simulink model "rocket"  (R2020a)
settings: Solver=FixedStepAuto  StartTime=0.0  StopTime=60  FixedStep=.1  RelTol=1e-3
InitFcn:
  | init
StopFcn:
  | plot_results
values from neighbouring files (symbols this model uses):
  d0 = 10    [init.m]
  d1 = 1    [init.m]
  F = 2*M*g    (= 21777.7777778)    [init.m]
  g = 9.8    [init.m]
  Ib = 1/4*mb*d1^2 + 1/12*mb*(2*d0)^2    (= 33583.3333333)    [init.m]
  M = mb + mc    (= 1111.11111111)    [init.m]
  mb = 1000    [init.m]
  mc = p/(1-p)*mb    (= 111.111111111)    [init.m]
  theta_ref = 10*pi/180    (= 0.174532925199)    [init.m]    (also in plot_results.m = out.theta_ref.Data)
libraries: simulink x2
settings Model: Creator=Tyler  LastModifiedBy=Tyler

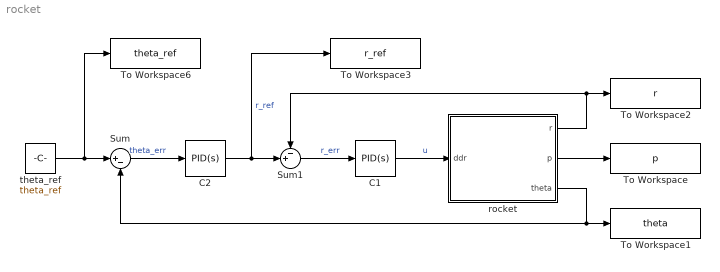
== system rocket ==
  C1 : simulink/Continuous/PID Controller  Controller=PID  Form=Parallel  TimeDomain=Continuous-time  UseExternalTs=off  SampleTime=-1  IntegratorMethod=Forward Euler  FilterMethod=Forward Euler  ControllerParametersSource=internal  P=30.7871197003863  I=15.2855535530538  D=10.7168713774137  UseFilter=on  N=29.8149109902028  TunerSelectOption=Transfer Function Based (PID Tuner App)  InitialConditionSource=internal  InitialConditionForIntegrator=0  InitialConditionForFilter=0  DifferentiatorICPrevScaledInput=0  ExternalReset=none  TrackingMode=off  Kt=1  LimitOutput=off  UpperSaturationLimit=inf  LowerSaturationLimit=-inf  LinearizeAsGain=on  AntiWindupMode=none  Kb=1  POutMin=[]  POutMax=[]  IOutMin=[]  IOutMax=[]  DOutMin=[]  DOutMax=[]  NOutMin=[]  NOutMax=[]  SumOutMin=[]  SumOutMax=[]  SaturationOutMin=[]  SaturationOutMax=[]  PParamMin=[]  PParamMax=[]  IParamMin=[]  IParamMax=[]  DParamMin=[]  DParamMax=[]  NParamMin=[]  NParamMax=[]  KbParamMin=[]  KbParamMax=[]  KtParamMin=[]  KtParamMax=[]  KbOutMin=[]  KbOutMax=[]  KtOutMin=[]  KtOutMax=[]  IntegratorOutMin=[]  IntegratorOutMax=[]  FilterOutMin=[]  FilterOutMax=[]  SumI1OutMin=[]  SumI1OutMax=[]  SumI2OutMin=[]  SumI2OutMax=[]  SumI3OutMin=[]  SumI3OutMax=[]  SumI4OutMin=[]  SumI4OutMax=[]  SumDOutMin=[]  SumDOutMax=[]  DifferentiatorOutMin=[]  DifferentiatorOutMax=[]  FilterDiffOutCoefMin=[]  FilterDiffOutCoefMax=[]  ReciprocalOutMin=[]  ReciprocalOutMax=[]  SumDenOutMin=[]  SumDenOutMax=[]  SumNumOutMin=[]  SumNumOutMax=[]  DivideOutMin=[]  DivideOutMax=[]  UdiffTsProdOutMin=[]  UdiffTsProdOutMax=[]  NTsProdOutMin=[]  NTsProdOutMax=[]  UintegralTsProdOutMin=[]  UintegralTsProdOutMax=[]  UngainTsProdOutMin=[]  UngainTsProdOutMax=[]  IntegratorContinuousStateAttributes=''  IntegratorStateMustResolveToSignalObject=off  IntegratorRTWStateStorageClass=Auto  FilterContinuousStateAttributes=''  FilterStateMustResolveToSignalObject=off  FilterRTWStateStorageClass=Auto  ParallelPVariant=InternalParameters  IdealPVariant=Disabled  IVariant=InternalParameters  DVariant=InternalParameters  IntegratorVariant=Continuous  SatVariant=Disabled  AWVariant=Passthrough  PCopyVariant=Disabled  TRVariant=Disabled  FdbkBlocksVariant=Forward  IdealPFdbkVariant=Disabled  SatFdbkVariant=Disabled  DerivativeFilterVariant=ContFilter  NVariant=InternalParameters  NCopyVariant=Disabled  FilterICVariant=InternalICsFilter  IntegratorICVariant=InternalICs  ExternalResetVariant=Disabled  TRSumVariant=Passthrough  SumFdbkVariant=Disabled  SumVariant=Sum_PID  TsampFilterVariant=InternalTs  TsampNgainVariant=Passthrough  TsampIntegralVariant=Passthrough
  C2 : simulink/Continuous/PID Controller  Controller=PID  Form=Parallel  TimeDomain=Continuous-time  UseExternalTs=off  SampleTime=-1  IntegratorMethod=Forward Euler  FilterMethod=Forward Euler  ControllerParametersSource=internal  P=0.486154115731224  I=0.0253600241547768  D=2.20545552139545  UseFilter=on  N=2.12291335792304  TunerSelectOption=Transfer Function Based (PID Tuner App)  InitialConditionSource=internal  InitialConditionForIntegrator=0  InitialConditionForFilter=0  DifferentiatorICPrevScaledInput=0  ExternalReset=none  TrackingMode=off  Kt=1  LimitOutput=off  UpperSaturationLimit=inf  LowerSaturationLimit=-inf  LinearizeAsGain=on  AntiWindupMode=none  Kb=1  POutMin=[]  POutMax=[]  IOutMin=[]  IOutMax=[]  DOutMin=[]  DOutMax=[]  NOutMin=[]  NOutMax=[]  SumOutMin=[]  SumOutMax=[]  SaturationOutMin=[]  SaturationOutMax=[]  PParamMin=[]  PParamMax=[]  IParamMin=[]  IParamMax=[]  DParamMin=[]  DParamMax=[]  NParamMin=[]  NParamMax=[]  KbParamMin=[]  KbParamMax=[]  KtParamMin=[]  KtParamMax=[]  KbOutMin=[]  KbOutMax=[]  KtOutMin=[]  KtOutMax=[]  IntegratorOutMin=[]  IntegratorOutMax=[]  FilterOutMin=[]  FilterOutMax=[]  SumI1OutMin=[]  SumI1OutMax=[]  SumI2OutMin=[]  SumI2OutMax=[]  SumI3OutMin=[]  SumI3OutMax=[]  SumI4OutMin=[]  SumI4OutMax=[]  SumDOutMin=[]  SumDOutMax=[]  DifferentiatorOutMin=[]  DifferentiatorOutMax=[]  FilterDiffOutCoefMin=[]  FilterDiffOutCoefMax=[]  ReciprocalOutMin=[]  ReciprocalOutMax=[]  SumDenOutMin=[]  SumDenOutMax=[]  SumNumOutMin=[]  SumNumOutMax=[]  DivideOutMin=[]  DivideOutMax=[]  UdiffTsProdOutMin=[]  UdiffTsProdOutMax=[]  NTsProdOutMin=[]  NTsProdOutMax=[]  UintegralTsProdOutMin=[]  UintegralTsProdOutMax=[]  UngainTsProdOutMin=[]  UngainTsProdOutMax=[]  IntegratorContinuousStateAttributes=''  IntegratorStateMustResolveToSignalObject=off  IntegratorRTWStateStorageClass=Auto  FilterContinuousStateAttributes=''  FilterStateMustResolveToSignalObject=off  FilterRTWStateStorageClass=Auto  ParallelPVariant=InternalParameters  IdealPVariant=Disabled  IVariant=InternalParameters  DVariant=InternalParameters  IntegratorVariant=Continuous  SatVariant=Disabled  AWVariant=Passthrough  PCopyVariant=Disabled  TRVariant=Disabled  FdbkBlocksVariant=Forward  IdealPFdbkVariant=Disabled  SatFdbkVariant=Disabled  DerivativeFilterVariant=ContFilter  NVariant=InternalParameters  NCopyVariant=Disabled  FilterICVariant=InternalICsFilter  IntegratorICVariant=InternalICs  ExternalResetVariant=Disabled  TRSumVariant=Passthrough  SumFdbkVariant=Disabled  SumVariant=Sum_PID  TsampFilterVariant=InternalTs  TsampNgainVariant=Passthrough  TsampIntegralVariant=Passthrough
  Sum : Sum  Inputs=|+-
  Sum1 : Sum  Inputs=-+|
  To Workspace : ToWorkspace  VariableName=p  SaveFormat=Timeseries  SampleTime=-1
  To Workspace1 : ToWorkspace  VariableName=theta  SaveFormat=Timeseries  SampleTime=-1
  To Workspace2 : ToWorkspace  VariableName=r  SaveFormat=Timeseries  SampleTime=-1
  To Workspace3 : ToWorkspace  VariableName=r_ref  SaveFormat=Timeseries  SampleTime=-1
  To Workspace6 : ToWorkspace  VariableName=theta_ref  SaveFormat=Timeseries  SampleTime=-1
  rocket : Subsystem
  theta_ref : Constant  Value=theta_ref
  wires:
  Sum1/1 -> C1/1  "r_err"
  rocket/3(theta) -> To Workspace1/1, Sum/2
  C1/1 -> rocket/1(ddr)  "u"
  rocket/1(r) -> To Workspace2/1, Sum1/1
  rocket/2(p) -> To Workspace/1
  Sum/1 -> C2/1  "theta_err"
  C2/1 -> To Workspace3/1, Sum1/2  "r_ref"
  theta_ref/1 -> To Workspace6/1, Sum/1

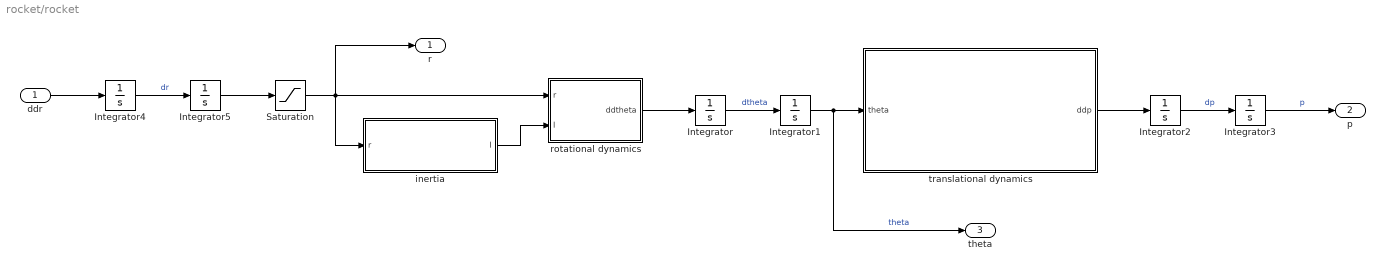
== system rocket/rocket ==
  ddr : Inport
  Integrator{,1..5} (6 alike) : Integrator
  Saturation : Saturate  UpperLimit=1  LowerLimit=-1
  inertia : Subsystem
  rotational dynamics : Subsystem
  translational dynamics : Subsystem
  r : Outport
  p : Outport  Port=2
  theta : Outport  Port=3
  wires:
  Integrator5/1 -> Saturation/1
  Integrator/1 -> Integrator1/1  "dtheta"
  inertia/1(I) -> rotational dynamics/2(I)
  rotational dynamics/1(ddtheta) -> Integrator/1
  Integrator4/1 -> Integrator5/1  "dr"
  Integrator2/1 -> Integrator3/1  "dp"
  Integrator3/1 -> p/1  "p"
  translational dynamics/1(ddp) -> Integrator2/1
  ddr/1 -> Integrator4/1
  Saturation/1 -> r/1, rotational dynamics/1(r), inertia/1(r)
  Integrator1/1 -> theta/1, translational dynamics/1(theta)  "theta"

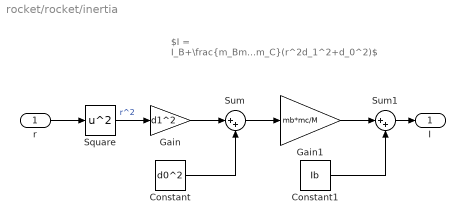
== system rocket/rocket/inertia ==
  note: $I = I_B+\frac{m_Bm_C}{m_B+m_C}(r^2d_1^2+d_0^2)$
  r : Inport
  Constant : Constant  Value=d0^2
  Constant1 : Constant  Value=Ib
  Gain : Gain  Gain=d1^2
  Gain1 : Gain  Gain=mb*mc/M
  Square : Math  Operator=square  SaturateOnIntegerOverflow=on
  Sum : Sum  Inputs=|++
  Sum1 : Sum  Inputs=|++
  I : Outport
  wires:
  Gain/1 -> Sum/1
  Gain1/1 -> Sum1/1
  Constant/1 -> Sum/2
  Constant1/1 -> Sum1/2
  Square/1 -> Gain/1  "r^2"
  Sum/1 -> Gain1/1
  r/1 -> Square/1
  Sum1/1 -> I/1

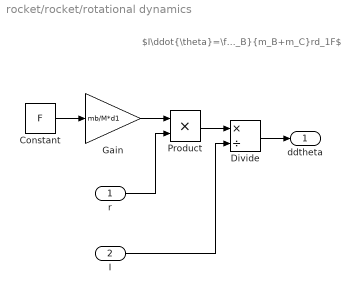
== system rocket/rocket/rotational dynamics ==
  note: $I\ddot{\theta}=\frac{m_B}{m_B+m_C}rd_1F$
  r : Inport
  I : Inport  Port=2
  Constant : Constant  Value=F
  Divide : Product  Inputs=*/
  Gain : Gain  Gain=mb/M*d1
  Product : Product
  ddtheta : Outport
  wires:
  Divide/1 -> ddtheta/1
  I/1 -> Divide/2
  Constant/1 -> Gain/1
  r/1 -> Product/2
  Product/1 -> Divide/1
  Gain/1 -> Product/1

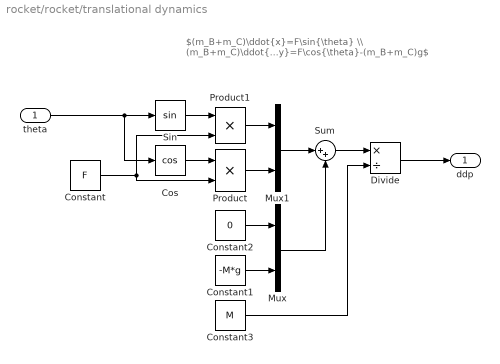
== system rocket/rocket/translational dynamics ==
  note: $(m_B+m_C)\ddot{x}=F\sin{\theta} \\ (m_B+m_C)\ddot{y}=F\cos{\theta}-(m_B+m_C)g$
  theta : Inport
  Constant : Constant  Value=F
  Constant1 : Constant  Value=-M*g
  Constant2 : Constant  Value=0
  Constant3 : Constant  Value=M
  Cos : Trigonometry  Operator=cos
  Divide : Product  Inputs=*/
  Mux : Mux  Inputs=2
  Mux1 : Mux  Inputs=2
  Product : Product
  Product1 : Product
  Sin : Trigonometry
  Sum : Sum  Inputs=|++
  ddp : Outport
  wires:
  Mux/1 -> Sum/2
  Sum/1 -> Divide/1
  Product1/1 -> Mux1/1
  Constant1/1 -> Mux/2
  theta/1 -> Cos/1, Sin/1
  Sin/1 -> Product1/1
  Divide/1 -> ddp/1
  Constant2/1 -> Mux/1
  Constant/1 -> Product1/2, Product/2
  Cos/1 -> Product/1
  Mux1/1 -> Sum/1
  Product/1 -> Mux1/2
  Constant3/1 -> Divide/2
